simulink model "DataSource"  (R2022b)
settings: Solver=VariableStepAuto  StartTime=0.0  StopTime=10.0  RelTol=1e-3
undefined symbols (not defined in the file or in its folder): Data, Preamble
libraries: hdlsllib x2
settings Model: Creator=Ceribro  LastModifiedBy=Ceribro

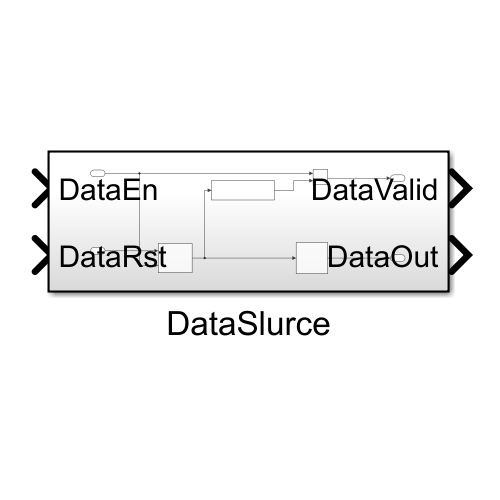
[thumbnail: Simulink's stored preview of the top-level diagram]
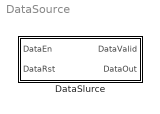
== system DataSource ==
  DataSlurce : Subsystem

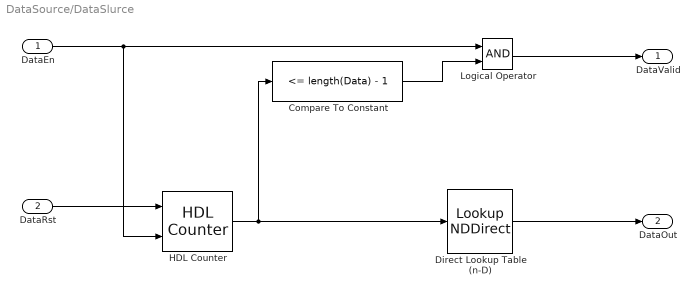
== system DataSource/DataSlurce ==
  DataEn : Inport
  DataRst : Inport  Port=2
  Compare To Constant : hdlsllib/Logic and Bit Operations/Compare To Constant  relop=<=  const=length(Data) - 1  OutDataTypeStr=boolean
  Direct Lookup Table (n-D) : LookupNDDirect  NumberOfTableDimensions=1  Table=[Preamble ]  DiagnosticForOutOfRangeInput=Error
  HDL Counter : hdlsllib/Sources/HDL Counter  CountType=Count limited  CountInit=0  CountStep=1  CountMax=length(Data) - 1  CountFromType=Initial value  CountFrom=0  CountResetPort=on  CountLoadPort=off  CountEnbPort=on  CountDirPort=off  CountHitOutputPort=off  CountDataType=Unsigned  CountWordLen=8  CountFracLen=0  CountSampTime=1
  Logical Operator : Logic  AllPortsSameDT=off  OutDataTypeStr=boolean
  DataValid : Outport
  DataOut : Outport  Port=2
  wires:
  HDL Counter/1 -> Compare To Constant/1, Direct Lookup Table (n-D)/1
  Compare To Constant/1 -> Logical Operator/2
  Logical Operator/1 -> DataValid/1
  DataRst/1 -> HDL Counter/1
  Direct Lookup Table (n-D)/1 -> DataOut/1
  DataEn/1 -> HDL Counter/2, Logical Operator/1
